simulink model "spring_damper"  (R2020b)
settings: Solver=VariableStepAuto  StartTime=0.0  StopTime=50.0  RelTol=1e-3
values from neighbouring files (symbols this model uses):
  b = 50    [variables.mat]
  k1 = 50    [variables.mat]
  k12 = 100    [variables.mat]
  M = 100    [variables.mat]
  m = 0.001    [variables.mat]
settings Model: Creator=JAGRUTI SHINDE  LastModifiedBy=JAGRUTI SHINDE

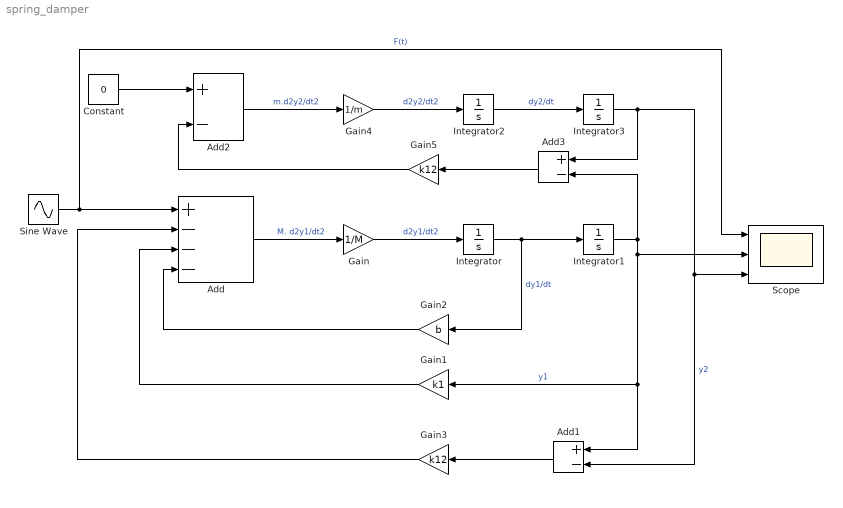
== system spring_damper ==
  Add : Sum  Inputs=+---
  Add1 : Sum  Inputs=+-
  Add2 : Sum  Inputs=+-
  Add3 : Sum  Inputs=+-
  Constant : Constant  Value=0
  Gain : Gain  Gain=1/M
  Gain1 : Gain  Gain=k1
  Gain2 : Gain  Gain=b
  Gain3 : Gain  Gain=k12
  Gain4 : Gain  Gain=1/m
  Gain5 : Gain  Gain=k12
  Integrator{,1..3} (4 alike) : Integrator
  Scope : Scope  NumInputPorts=3
  Sine Wave : Sin  Amplitude=2  Frequency=10  SampleTime=0
  wires:
  Add/1 -> Gain/1  "M. d2y1/dt2"
  Gain/1 -> Integrator/1  "d2y1/dt2"
  Integrator/1 -> Gain2/1, Integrator1/1  "dy1/dt"
  Integrator1/1 -> Add1/1, Gain1/1, Scope/2, Add3/2  "y1"
  Gain2/1 -> Add/4
  Gain1/1 -> Add/3
  Add1/1 -> Gain3/1
  Gain3/1 -> Add/2
  Add2/1 -> Gain4/1  "m.d2y2/dt2"
  Gain4/1 -> Integrator2/1  "d2y2/dt2"
  Integrator2/1 -> Integrator3/1  "dy2/dt"
  Integrator3/1 -> Add3/1, Scope/3, Add1/2  "y2"
  Add3/1 -> Gain5/1
  Gain5/1 -> Add2/2
  Constant/1 -> Add2/1
  Sine Wave/1 -> Scope/1, Add/1  "F(t)"
